simulink model "PDTest"  (R2014a)
settings: Solver=ode45  StartTime=0.0  StopTime=10.0  RelTol=1e-3
values from neighbouring files (symbols this model uses):
  C = [1 0 0 0 0 0;0 0 1 0 0 0;0 0 0 0 1 0]    [parameters1.m]
  I = 1/12*m*((2*ry1)^2 + (2*rx1)^2)    (= 7.53502955357)    [parameters1.m]
  k1m = 50    [parameters1.m]
  k1x = 100    [parameters1.m]
  k1y = 100    [parameters1.m]
  k2m = 25    [parameters1.m]
  k2x = 60    [parameters1.m]
  k2y = 60    [parameters1.m]
undefined symbols (not defined in the file): m
libraries: simulink x3
settings Model: Creator=propagator  LastModifiedBy=propagator
settings OptimizationCC: SimCompilerOptimization=On
settings HardwareCC: ProdBitPerLong=64  ProdBitPerPointer=64  ProdIntDivRoundTo=Zero  ProdEndianess=LittleEndian  ProdWordSize=64  ProdHWDeviceType=Intel->x86-64
settings ModelReferenceCC: EnableParallelModelReferenceBuilds=on
settings RTWCC: BuildConfiguration=Faster Runs  TargetLang=C++
settings GRTTargetCC: MultiInstanceERTCode=on  CodeInterfacePackaging=C++ class

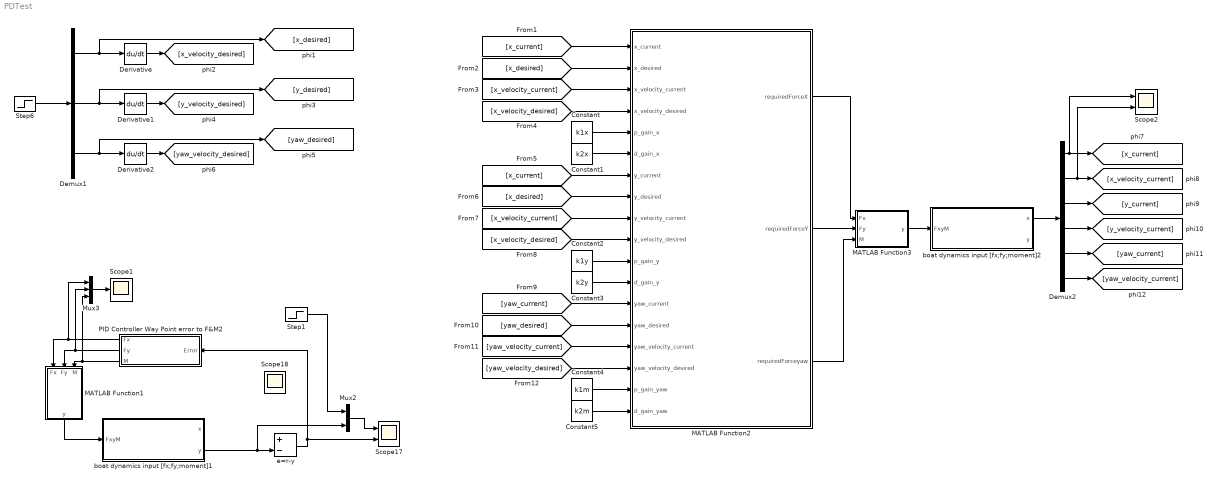
== system PDTest ==
  Constant : Constant  Value=k1x
  Constant1 : Constant  Value=k2x
  Constant2 : Constant  Value=k1y
  Constant3 : Constant  Value=k2y
  Constant4 : Constant  Value=k1m
  Constant5 : Constant  Value=k2m
  Demux1 : Demux  Outputs=3
  Demux2 : Demux  Outputs=6
  Derivative : Derivative
  Derivative1 : Derivative
  Derivative2 : Derivative
  MATLAB Function1 : MATLAB Function  TreatAsAtomicUnit=on
  MATLAB Function2 : MATLAB Function  TreatAsAtomicUnit=on
  MATLAB Function3 : MATLAB Function  TreatAsAtomicUnit=on
  Mux2 : Mux  Inputs=2
  Mux3 : Mux  Inputs=3
  PID Controller Way Point error to F&M2 : Subsystem
  Scope1 : Scope
      settings: YMin=-0.014  YMax=0  SaveName=ScopeData4
  Scope17 : Scope  NumInputPorts=2
      settings: YMin=0~0  YMax=70~17
  Scope18 : Scope
      settings: SaveName=ScopeData2
  Scope2 : Scope  NumInputPorts=2
      settings: YMin=0~0  YMax=70~17  SaveName=ScopeData3
  Step1 : Step  Before=[0;0;0]  After=[10;0;0]  SampleTime=0
  Step6 : Step  Before=[0;0;0]  After=[10;0;0]  SampleTime=0
  boat dynamics input [fx;fy;moment]1 : Subsystem  mask{M=m, I=I, fw=0, kr=0, C=C}
      mask prompts: M "Mass"; I "Inert"; fw "Water Friction"; kr "Rotational water Friction"; C "Output Matrix"
  boat dynamics input [fx;fy;moment]2 : Subsystem  mask{M=m, I=I, fw=0, kr=0, C=C}
      mask prompts: M "Mass"; I "Inert"; fw "Water Friction"; kr "Rotational water Friction"; C "Output Matrix"
  e=r-y : Sum  Inputs=+-
  wires:
  e=r-y/1 -> PID Controller Way Point error to F&M2/1(Error), Scope17/2
  PID Controller Way Point error to F&M2/1(Fx) -> Mux3/1, MATLAB Function1/1(Fx)
  MATLAB Function1/1(y) -> boat dynamics input [fx;fy;moment]1/1(FxyM)
  PID Controller Way Point error to F&M2/2(Fy) -> Mux3/2, MATLAB Function1/2(Fy)
  PID Controller Way Point error to F&M2/3(M) -> Mux3/3, MATLAB Function1/3(M)
  boat dynamics input [fx;fy;moment]1/2(y) -> Mux2/2, e=r-y/2
  Mux2/1 -> Scope17/1
  MATLAB Function3/1(y) -> boat dynamics input [fx;fy;moment]2/1(FxyM)
  boat dynamics input [fx;fy;moment]2/1(x) -> Demux2/1
  Demux2/1 -> Scope2/1, [x_current]
  Demux2/3 -> [y_current]
  Demux2/4 -> [y_velocity_current]
  Demux2/5 -> [yaw_current]
  Demux2/6 -> [yaw_velocity_current]
  Mux3/1 -> Scope1/1
  Step1/1 -> Mux2/1
  MATLAB Function2/1(requiredForceX) -> MATLAB Function3/1(Fx)
  MATLAB Function2/2(requiredForceY) -> MATLAB Function3/2(Fy)
  MATLAB Function2/3(requiredForceyaw) -> MATLAB Function3/3(M)
  [x_desired] -> MATLAB Function2/8(y_desired)
  [x_velocity_current] -> MATLAB Function2/9(y_velocity_current)
  [yaw_current] -> MATLAB Function2/13(yaw_current)
  [x_velocity_desired] -> MATLAB Function2/10(y_velocity_desired)
  [yaw_desired] -> MATLAB Function2/14(yaw_desired)
  [yaw_velocity_current] -> MATLAB Function2/15(yaw_velocity_current)
  [yaw_velocity_desired] -> MATLAB Function2/16(yaw_velocity_desired)
  [x_velocity_desired] -> MATLAB Function2/4(x_velocity_desired)
  [x_current] -> MATLAB Function2/7(y_current)
  [x_velocity_current] -> MATLAB Function2/3(x_velocity_current)
  [x_desired] -> MATLAB Function2/2(x_desired)
  [x_current] -> MATLAB Function2/1(x_current)
  Constant2/1 -> MATLAB Function2/11(p_gain_y)
  Constant3/1 -> MATLAB Function2/12(d_gain_y)
  Constant5/1 -> MATLAB Function2/18(d_gain_yaw)
  Constant4/1 -> MATLAB Function2/17(p_gain_yaw)
  Constant/1 -> MATLAB Function2/5(p_gain_x)
  Constant1/1 -> MATLAB Function2/6(d_gain_x)
  Demux2/2 -> Scope2/2, [x_velocity_current]
  Derivative2/1 -> [yaw_velocity_desired]
  Demux1/3 -> [yaw_desired], Derivative2/1
  Step6/1 -> Demux1/1
  Derivative/1 -> [x_velocity_desired]
  Derivative1/1 -> [y_velocity_desired]
  Demux1/1 -> [x_desired], Derivative/1
  Demux1/2 -> [y_desired], Derivative1/1

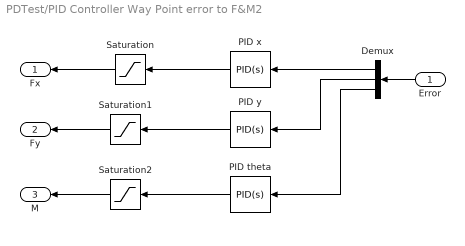
== system PDTest/PID Controller Way Point error to F&M2 ==
  Error : Inport
  Demux : Demux  Outputs=3
  PID theta : simulink/Continuous/PID Controller  Controller=PID  TimeDomain=Continuous-time  SampleTime=1  IntegratorMethod=Forward Euler  FilterMethod=Forward Euler  Form=Parallel  P=k1m  I=0  D=k2m  N=3.646824066771  InitialConditionSource=internal  InitialConditionForIntegrator=0  InitialConditionForFilter=0  ExternalReset=none  LimitOutput=off  UpperSaturationLimit=inf  LowerSaturationLimit=-inf  LinearizeAsGain=off  AntiWindupMode=none  Kb=1  TrackingMode=off  Kt=1  PParamMin=[]  PParamMax=[]  IParamMin=[]  IParamMax=[]  DParamMin=[]  DParamMax=[]  NParamMin=[]  NParamMax=[]  KbParamMin=[]  KbParamMax=[]  KtParamMin=[]  KtParamMax=[]  POutMin=[]  POutMax=[]  IOutMin=[]  IOutMax=[]  DOutMin=[]  DOutMax=[]  NOutMin=[]  NOutMax=[]  KbOutMin=[]  KbOutMax=[]  KtOutMin=[]  KtOutMax=[]  IntegratorOutMin=[]  IntegratorOutMax=[]  FilterOutMin=[]  FilterOutMax=[]  SumOutMin=[]  SumOutMax=[]  SumI1OutMin=[]  SumI1OutMax=[]  SumI2OutMin=[]  SumI2OutMax=[]  SumI3OutMin=[]  SumI3OutMax=[]  SumDOutMin=[]  SumDOutMax=[]  SaturationOutMin=[]  SaturationOutMax=[]  IntegratorContinuousStateAttributes=''  IntegratorStateMustResolveToSignalObject=off  IntegratorRTWStateStorageClass=Auto  FilterContinuousStateAttributes=''  FilterStateMustResolveToSignalObject=off  FilterRTWStateStorageClass=Auto
  PID x : simulink/Continuous/PID Controller  Controller=PID  TimeDomain=Continuous-time  SampleTime=1  IntegratorMethod=Forward Euler  FilterMethod=Forward Euler  Form=Parallel  P=k1x  I=0  D=k2x  N=3.646824066771  InitialConditionSource=internal  InitialConditionForIntegrator=0  InitialConditionForFilter=0  ExternalReset=none  LimitOutput=off  UpperSaturationLimit=inf  LowerSaturationLimit=-inf  LinearizeAsGain=off  AntiWindupMode=none  Kb=1  TrackingMode=off  Kt=1  PParamMin=[]  PParamMax=[]  IParamMin=[]  IParamMax=[]  DParamMin=[]  DParamMax=[]  NParamMin=[]  NParamMax=[]  KbParamMin=[]  KbParamMax=[]  KtParamMin=[]  KtParamMax=[]  POutMin=[]  POutMax=[]  IOutMin=[]  IOutMax=[]  DOutMin=[]  DOutMax=[]  NOutMin=[]  NOutMax=[]  KbOutMin=[]  KbOutMax=[]  KtOutMin=[]  KtOutMax=[]  IntegratorOutMin=[]  IntegratorOutMax=[]  FilterOutMin=[]  FilterOutMax=[]  SumOutMin=[]  SumOutMax=[]  SumI1OutMin=[]  SumI1OutMax=[]  SumI2OutMin=[]  SumI2OutMax=[]  SumI3OutMin=[]  SumI3OutMax=[]  SumDOutMin=[]  SumDOutMax=[]  SaturationOutMin=[]  SaturationOutMax=[]  IntegratorContinuousStateAttributes=''  IntegratorStateMustResolveToSignalObject=off  IntegratorRTWStateStorageClass=Auto  FilterContinuousStateAttributes=''  FilterStateMustResolveToSignalObject=off  FilterRTWStateStorageClass=Auto
  PID y : simulink/Continuous/PID Controller  Controller=PID  TimeDomain=Continuous-time  SampleTime=1  IntegratorMethod=Forward Euler  FilterMethod=Forward Euler  Form=Parallel  P=k1y  I=0  D=k2y  N=4  InitialConditionSource=internal  InitialConditionForIntegrator=0  InitialConditionForFilter=0  ExternalReset=none  LimitOutput=off  UpperSaturationLimit=inf  LowerSaturationLimit=-inf  LinearizeAsGain=off  AntiWindupMode=none  Kb=1  TrackingMode=off  Kt=1  PParamMin=[]  PParamMax=[]  IParamMin=[]  IParamMax=[]  DParamMin=[]  DParamMax=[]  NParamMin=[]  NParamMax=[]  KbParamMin=[]  KbParamMax=[]  KtParamMin=[]  KtParamMax=[]  POutMin=[]  POutMax=[]  IOutMin=[]  IOutMax=[]  DOutMin=[]  DOutMax=[]  NOutMin=[]  NOutMax=[]  KbOutMin=[]  KbOutMax=[]  KtOutMin=[]  KtOutMax=[]  IntegratorOutMin=[]  IntegratorOutMax=[]  FilterOutMin=[]  FilterOutMax=[]  SumOutMin=[]  SumOutMax=[]  SumI1OutMin=[]  SumI1OutMax=[]  SumI2OutMin=[]  SumI2OutMax=[]  SumI3OutMin=[]  SumI3OutMax=[]  SumDOutMin=[]  SumDOutMax=[]  SaturationOutMin=[]  SaturationOutMax=[]  IntegratorContinuousStateAttributes=''  IntegratorStateMustResolveToSignalObject=off  IntegratorRTWStateStorageClass=Auto  FilterContinuousStateAttributes=''  FilterStateMustResolveToSignalObject=off  FilterRTWStateStorageClass=Auto
  Saturation : Saturate  UpperLimit=100  LowerLimit=-100
  Saturation1 : Saturate  UpperLimit=100  LowerLimit=-100
  Saturation2 : Saturate  UpperLimit=50  LowerLimit=-50
  Fx : Outport
  Fy : Outport  Port=2
  M : Outport  Port=3
  wires:
  Demux/1 -> PID x/1
  Demux/2 -> PID y/1
  Demux/3 -> PID theta/1
  Error/1 -> Demux/1
  PID x/1 -> Saturation/1
  Saturation/1 -> Fx/1
  PID y/1 -> Saturation1/1
  Saturation1/1 -> Fy/1
  PID theta/1 -> Saturation2/1
  Saturation2/1 -> M/1

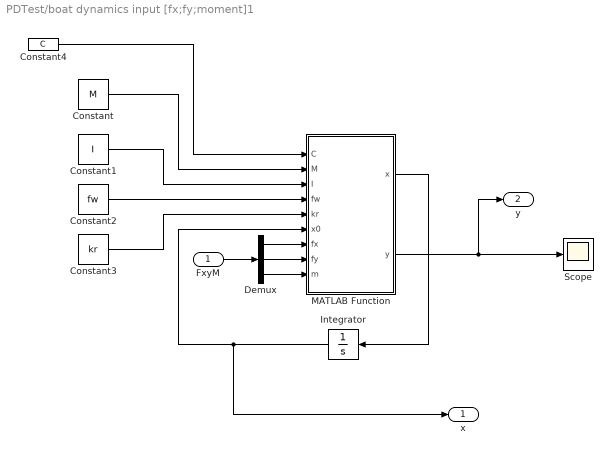
== system PDTest/boat dynamics input [fx;fy;moment]1 ==
  FxyM : Inport
  Constant : Constant  Value=M
  Constant1 : Constant  Value=I
  Constant2 : Constant  Value=fw
  Constant3 : Constant  Value=kr
  Constant4 : Constant  Value=C
  Demux : Demux  Outputs=3
  Integrator : Integrator  InitialCondition=[0 0 0 0 0 0]
  MATLAB Function : MATLAB Function  TreatAsAtomicUnit=on
  Scope : Scope
  x : Outport
  y : Outport  Port=2
  wires:
  MATLAB Function/2(y) -> Scope/1, y/1
  Integrator/1 -> x/1, MATLAB Function/6(x0)
  Constant/1 -> MATLAB Function/2(M)
  Constant1/1 -> MATLAB Function/3(I)
  Constant2/1 -> MATLAB Function/4(fw)
  Constant3/1 -> MATLAB Function/5(kr)
  Constant4/1 -> MATLAB Function/1(C)
  MATLAB Function/1(x) -> Integrator/1
  FxyM/1 -> Demux/1
  Demux/1 -> MATLAB Function/7(fx)
  Demux/2 -> MATLAB Function/8(fy)
  Demux/3 -> MATLAB Function/9(m)

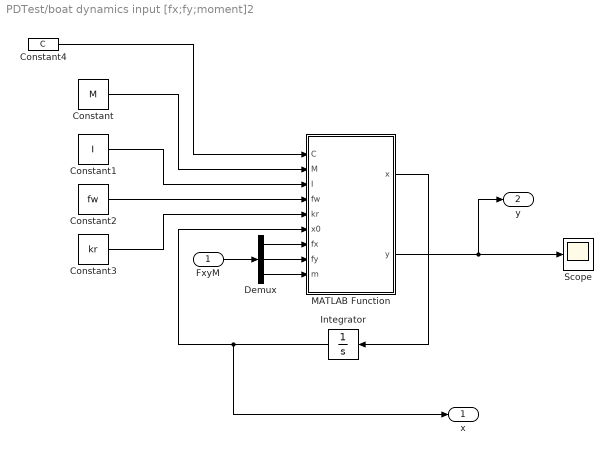
== system PDTest/boat dynamics input [fx;fy;moment]2 ==
  FxyM : Inport
  Constant : Constant  Value=M
  Constant1 : Constant  Value=I
  Constant2 : Constant  Value=fw
  Constant3 : Constant  Value=kr
  Constant4 : Constant  Value=C
  Demux : Demux  Outputs=3
  Integrator : Integrator  InitialCondition=[0 0 0 0 0 0]
  MATLAB Function : MATLAB Function  TreatAsAtomicUnit=on
  Scope : Scope
  x : Outport
  y : Outport  Port=2
  wires:
  MATLAB Function/2(y) -> Scope/1, y/1
  Integrator/1 -> x/1, MATLAB Function/6(x0)
  Constant/1 -> MATLAB Function/2(M)
  Constant1/1 -> MATLAB Function/3(I)
  Constant2/1 -> MATLAB Function/4(fw)
  Constant3/1 -> MATLAB Function/5(kr)
  Constant4/1 -> MATLAB Function/1(C)
  MATLAB Function/1(x) -> Integrator/1
  FxyM/1 -> Demux/1
  Demux/1 -> MATLAB Function/7(fx)
  Demux/2 -> MATLAB Function/8(fy)
  Demux/3 -> MATLAB Function/9(m)

== matlab function PDTest/MATLAB Function2 ==
  data: x_current input; requiredForceX output; x_desired input; x_velocity_current input; x_velocity_desired input; p_gain_x input; d_gain_x input; y_current input; y_desired input; y_velocity_current input; y_velocity_desired input; p_gain_y input; d_gain_y input; yaw_current input; yaw_desired input; yaw_velocity_current input; yaw_velocity_desired input; p_gain_yaw input; d_gain_yaw input; requiredForceY output; requiredForceyaw output
function [requiredForceX,requiredForceY,requiredForceyaw] = fcn(x_current,x_desired,x_velocity_current,x_velocity_desired, p_gain_x,d_gain_x,...
                            y_current,y_desired,y_velocity_current,y_velocity_desired, p_gain_y, d_gain_y,...
                            yaw_current,yaw_desired,yaw_velocity_current,yaw_velocity_desired, p_gain_yaw, d_gain_yaw)

requiredForceX = p_gain_x * (x_desired - x_current) + d_gain_x * (x_velocity_desired - x_velocity_current);
requiredForceY = p_gain_y * (y_desired - y_current) + d_gain_y * (y_velocity_desired - y_velocity_current);
requiredForceyaw = p_gain_yaw * (yaw_desired - yaw_current) + d_gain_yaw * (yaw_velocity_desired - yaw_velocity_current);
end

== matlab function PDTest/MATLAB Function3 ==
  data: Fx input; y output; Fy input; M input
function y = fcn(Fx,Fy,M)
%#codegen

y = [Fx;Fy;M];

== matlab function PDTest/boat dynamics input [fx;fy;moment]2/MATLAB Function ==
  data: C input; x output; M input; I input; fw input; kr input; x0 input; fx input; y output; fy input; m input
function [x,y] = systemstep(C,M,I,fw,kr,x0,fx,fy,m)

   % status vector y=[x;x_dot;y;_y_dot;theta;theta_dot]
   % forces u=[fx;fy;m]
   % contant parameters {mass; rotational inertia; friction coefficients }
   
   x1 = x0(2);
   x2 = fx/M - 0*x0(2)*fw;
   x3 = x0(4);
   x4 = fy/M - 0*x0(4)*fw;
   x5 = x0(6);
   x6 = m/I - 0*x0(6)*kr;

   x=[x1;x2;x3;x4;x5;x6];
   
   y = C*x0;

== matlab function PDTest/MATLAB Function1 ==
  data: Fx input; y output; Fy input; M input
function y = fcn(Fx,Fy,M)
%#codegen

y = [Fx;Fy;M];

== matlab function PDTest/boat dynamics input [fx;fy;moment]1/MATLAB Function ==
  data: C input; x output; M input; I input; fw input; kr input; x0 input; fx input; y output; fy input; m input
function [x,y] = systemstep(C,M,I,fw,kr,x0,fx,fy,m)

   % status vector y=[x;x_dot;y;_y_dot;theta;theta_dot]
   % forces u=[fx;fy;m]
   % contant parameters {mass; rotational inertia; friction coefficients }
   
   x1 = x0(2);
   x2 = fx/M - 0*x0(2)*fw;
   x3 = x0(4);
   x4 = fy/M - 0*x0(4)*fw;
   x5 = x0(6);
   x6 = m/I - 0*x0(6)*kr;

   x=[x1;x2;x3;x4;x5;x6];
   
   y = C*x0;
